simulink model "TST_DoorsRequirementsWithSurrogate"  (Simulink 10.0)
settings: Solver=FixedStepDiscrete  StartTime=0.0  StopTime=10.0  FixedStep=0.02  RelTol=1e-3  EnableMultiTasking=on
settings Model: reqMgrSettings="100 S'doors','misc'{{S'surrogatepath','savemodel','savesurrogate','updateLinks','doorsLinks2sl','slLinks2Doors','purgeDoors','purgeSimulink','detaillevel','surrogateId','synctime'{{T\"/Orion/Design/Air Vehicle Segment/Integrated Flight System/ToolTestbed/TST_DoorsRequirementsWithSurrogate\",M[1],M[1],M[0],M[0],M[0],M[0],M[0],M[4],T\"00000366\",T\"\"}},S'mode','pathStorage'{{T\"generic\",T\"modelRelative\"}}}}"  Creator=kharthforeign  LastModifiedBy=unknown
settings DataIOCC: LimitDataPoints=on  SignalLoggingSaveFormat=ModelDataLogs  SaveOutput=off  SignalLogging=off  SaveTime=off
settings OptimizationCC: BlockReduction=off  ConditionallyExecuteInputs=off  OptimizeBlockIOStorage=off  BufferReuse=off  GlobalBufferReuse=off  ExpressionFolding=off  ExpressionDepthLimit=2147483647  LocalBlockOutputs=off  InitFltsAndDblsToZero=on  OptimizeDataStoreBuffers=off  BusAssignmentInplaceUpdate=off
settings DebuggingCC: SolverPrmCheckMsg=warning  FcnCallInpInsideContextMsg=warning  StateNameClashWarn=warning
settings GRTTargetCC: GeneratePreprocessorConditionals=Disable all
settings ConfigComp: CovExternalEMLEnable=off

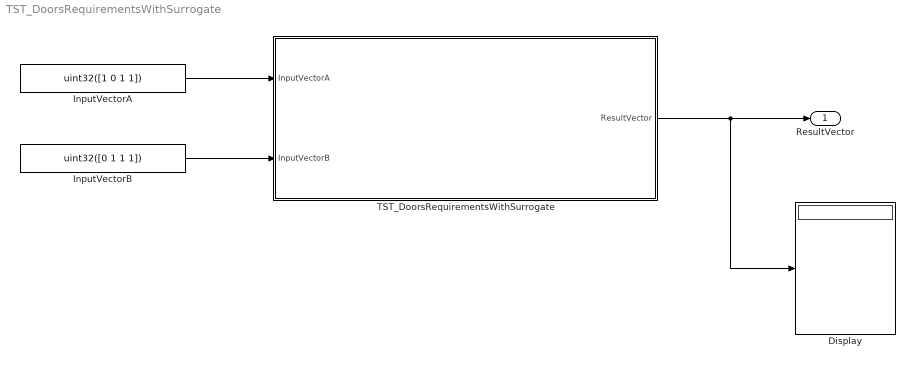
== system TST_DoorsRequirementsWithSurrogate ==
  Display : Display
  InputVectorA : Constant  Value=uint32([1 0 1 1])
  InputVectorB : Constant  Value=uint32([0 1 1 1])
  TST_DoorsRequirementsWithSurrogate : Subsystem  RequirementInfo={} %GIDa_611058af_54f9_4307_b99e_3d68e731bf77  TreatAsAtomicUnit=on
  ResultVector : Outport
  wires:
  TST_DoorsRequirementsWithSurrogate/1(ResultVector) -> ResultVector/1, Display/1
  InputVectorA/1 -> TST_DoorsRequirementsWithSurrogate/1(InputVectorA)
  InputVectorB/1 -> TST_DoorsRequirementsWithSurrogate/2(InputVectorB)

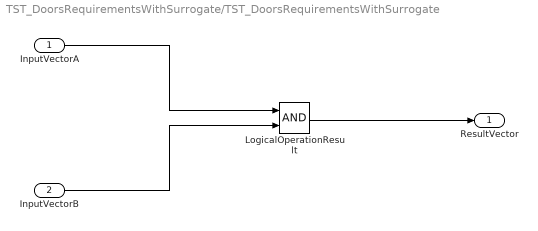
== system TST_DoorsRequirementsWithSurrogate/TST_DoorsRequirementsWithSurrogate ==
  InputVectorA : Inport
  InputVectorB : Inport  Port=2
  LogicalOperationResult : Logic  RequirementInfo={} %GIDa_cd8a7865_673e_4392_a46c_99735584f465  AllPortsSameDT=off  OutDataTypeStr=boolean
  ResultVector : Outport
  wires:
  InputVectorA/1 -> LogicalOperationResult/1
  InputVectorB/1 -> LogicalOperationResult/2
  LogicalOperationResult/1 -> ResultVector/1
